simulink model "Temp_derating"  (R2021b)
settings: Solver=VariableStepAuto  StartTime=0.0  StopTime=600  RelTol=1e-3
undefined symbols (not defined in the file): sigbuilder_block
settings Model: Creator=mohamednasser  LastModifiedBy=mohamednasser

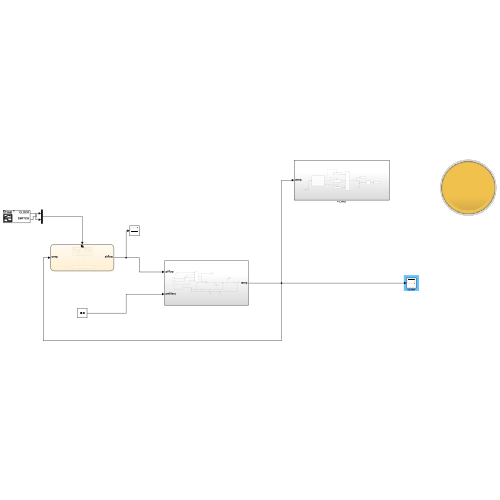
[thumbnail: Simulink's stored preview of the top-level diagram]
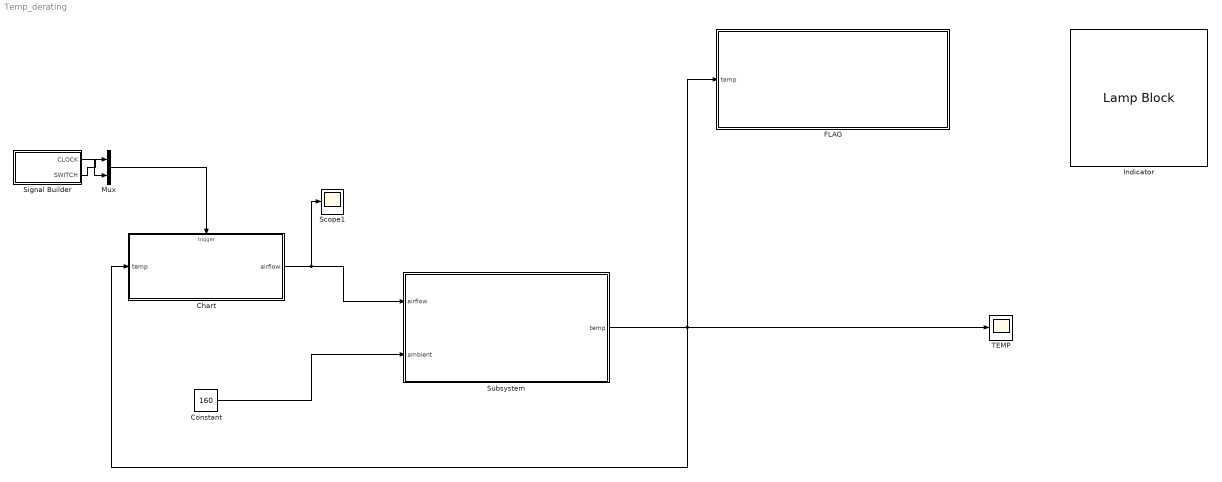
== system Temp_derating ==
  Chart : Stateflow chart  TreatAsAtomicUnit=on
  Constant : Constant  Value=160
  FLAG : Subsystem
  Indicator : LampBlock  LabelPosition=Hide
  Mux : Mux  Inputs=2
  Scope1 : Scope
  Signal Builder : Subsystem  Tag=STV Subsys  LoadFcn=sigbuilder_block('load');  StartFcn=sigbuilder_block('start');  StopFcn=sigbuilder_block('stop');  ClipboardFcn=sigbuilder_block('clipboard');  mask(Sigbuilder block){tuvar=[0:10]}
      mask help: Simulink:masks:SigbuilderBlock_MD
      mask init:
      | if ~strcmp(get_param(bdroot(gcbh),'SimulationStatus'),'stopped') tuvar = sigbuilder_block('maskInit'); end
      settings: CopyFcn=sigbuilder_block('copy');  DeleteFcn=sigbuilder_block('delete');  ModelCloseFcn=sigbuilder_block('modelClose');  PreSaveFcn=sigbuilder_block('preSave');  PauseFcn=sigbuilder_block('pause');  ContinueFcn=sigbuilder_block('continue');  NameChangeFcn=sigbuilder_block('namechange');  OpenFcn=sigbuilder_block('open',[377 114 550 400 ]);  CloseFcn=sigbuilder_block('close');
      mask Display: plot(0, 0, 100, 100,[2, 2, 32, 32, 2], [68, 8, 8, 68, 68],[32, 2], [38, 38], [32, 19, 2],[53, 60, 44], [32, 17, 17, 2],[16, 16, 31, 31]);txt = getActiveGroup(gcbh);text(2, 100, txt,'verticalAlignment', 'top');
  Subsystem : Subsystem
  TEMP : Scope
  wires:
  Subsystem/1(temp) -> TEMP/1, FLAG/1(temp), Chart/1(temp)
  Constant/1 -> Subsystem/2(ambient)
  Chart/1(airflow) -> Scope1/1, Subsystem/1(airflow)
  Mux/1 -> Chart/Trigger
  Signal Builder/1(CLOCK) -> Mux/2
  Signal Builder/2(SWITCH) -> Mux/1

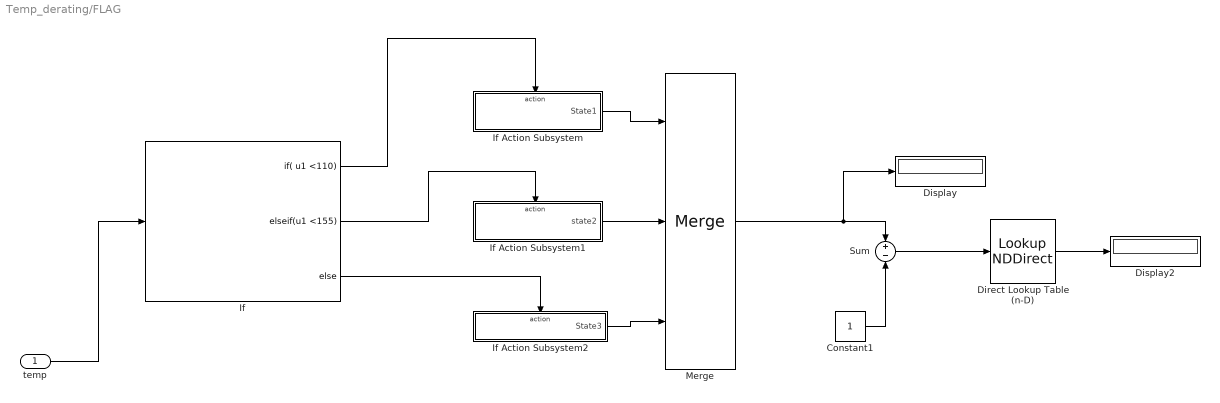
== system Temp_derating/FLAG ==
  temp : Inport
  Constant1 : Constant
  Direct Lookup Table (n-D) : LookupNDDirect  NumberOfTableDimensions=1  Table=[1 2 3]
  Display : Display
  Display2 : Display
  If : If  IfExpression=u1 <110  ElseIfExpressions=u1 <155
  If Action Subsystem : Subsystem  TreatAsAtomicUnit=on
  If Action Subsystem1 : Subsystem  TreatAsAtomicUnit=on
  If Action Subsystem2 : Subsystem  TreatAsAtomicUnit=on
  Merge : Merge  Inputs=3
  Sum : Sum  Inputs=+-
  wires:
  If/2 -> If Action Subsystem1/Action
  If/1 -> If Action Subsystem/Action
  Constant1/1 -> Sum/2
  Merge/1 -> Display/1, Sum/1
  If/3 -> If Action Subsystem2/Action
  If Action Subsystem1/1(state2) -> Merge/2
  Sum/1 -> Direct Lookup Table (n-D)/1
  If Action Subsystem/1(State1) -> Merge/1
  temp/1 -> If/1
  If Action Subsystem2/1(State3) -> Merge/3
  Direct Lookup Table (n-D)/1 -> Display2/1

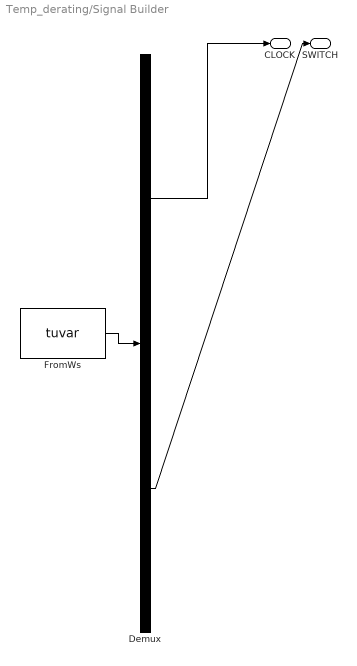
== system Temp_derating/Signal Builder ==
  Demux : Demux  Tag=STV Demux  Outputs=2
      settings: DisplayOption=none
  FromWs : FromWorkspace  Tag=STV FromWs  VariableName=tuvar
      SigBuilderData=|
      | common.afterFinalStr = 'Extrapolate'
      | common.sampleTime = 0
      | dataSet.timeRange = [0 600]
      | dataSet.name = 'Group 1'
      | sbobj.Groups.Name = 'Group 1'
      | sbobj.Groups.Signals(1).Name = 'CLOCK'
      | sbobj.Groups.Signals(1).XData = [0 0.5 0.5 1 1 1.5 1.5 2 2 2.5 2.5 3 ... (2400 elements, 1x2400)]
      | sbobj.Groups.Signals(1).YData = [2 2 0 0 2 2 0 0 2 2 0 0 ... (2400 elements, 1x2400)]
      | sbobj.Groups.Signals(2).Name = 'SWITCH'
      | sbobj.Groups.Signals(2).XData = [0 350 350 501 501 600]
      | sbobj.Groups.Signals(2).YData = [0 0 1 1 0 0]
      | sbobj.Groups.TimeRange = [0 600]
  CLOCK : Outport  Tag=STV Outport
  SWITCH : Outport  Tag=STV Outport  Port=2
  wires:
  FromWs/1 -> Demux/1
  Demux/1 -> CLOCK/1
  Demux/2 -> SWITCH/1

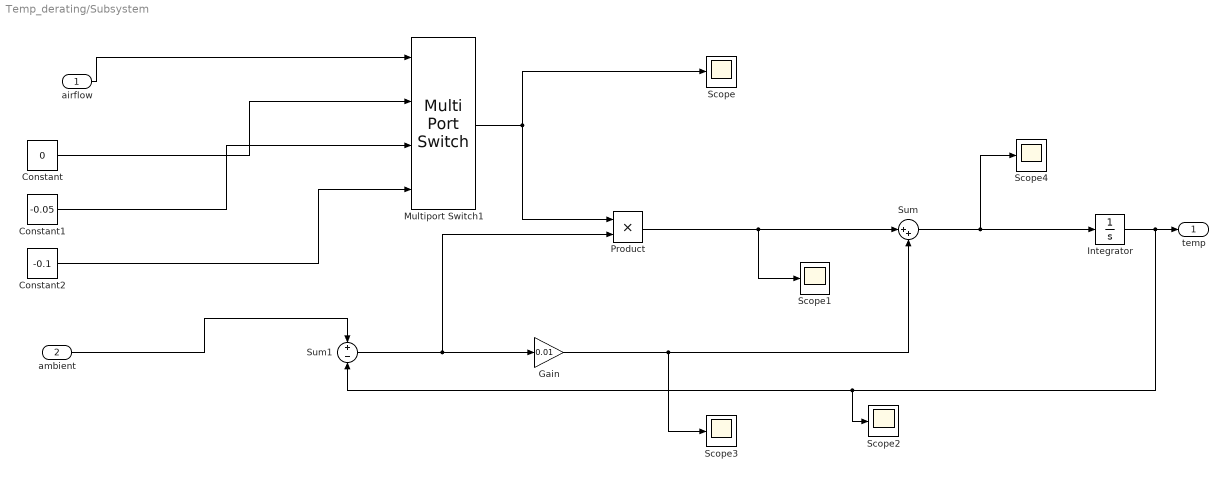
== system Temp_derating/Subsystem ==
  airflow : Inport
  ambient : Inport  Port=2
  Constant : Constant  Value=0
  Constant1 : Constant  Value=-0.05
  Constant2 : Constant  Value=-0.1
  Gain : Gain  Gain=0.01
  Integrator : Integrator  InitialCondition=70
  Multiport Switch1 : MultiPortSwitch  DataPortOrder=Zero-based contiguous  zeroidx=on
  Product : Product
  Scope{,1..4} (5 alike) : Scope
  Sum : Sum  Inputs=|++
  Sum1 : Sum  Inputs=+-
  temp : Outport
  wires:
  Constant/1 -> Multiport Switch1/2
  Constant2/1 -> Multiport Switch1/4
  airflow/1 -> Multiport Switch1/1
  Multiport Switch1/1 -> Product/1, Scope/1
  Constant1/1 -> Multiport Switch1/3
  ambient/1 -> Sum1/1
  Sum1/1 -> Product/2, Gain/1
  Sum/1 -> Scope4/1, Integrator/1
  Gain/1 -> Scope3/1, Sum/2
  Product/1 -> Scope1/1, Sum/1
  Integrator/1 -> Scope2/1, Sum1/2, temp/1

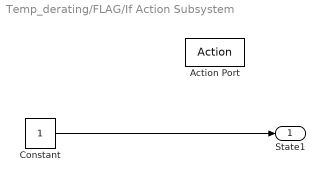
== system Temp_derating/FLAG/If Action Subsystem ==
  Action Port : ActionPort  ActionPortLabel=if( u1 <110)
  Constant : Constant
  State1 : Outport
  wires:
  Constant/1 -> State1/1

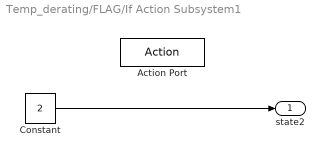
== system Temp_derating/FLAG/If Action Subsystem1 ==
  Action Port : ActionPort  ActionPortLabel=elseif(u1 <155)
  Constant : Constant  Value=2
  state2 : Outport
  wires:
  Constant/1 -> state2/1

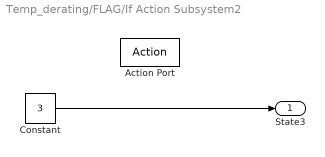
== system Temp_derating/FLAG/If Action Subsystem2 ==
  Action Port : ActionPort  ActionPortLabel=else
  Constant : Constant  Value=3
  State3 : Outport
  wires:
  Constant/1 -> State3/1

== stateflow chart Temp_derating/Chart ==
  settings: executeAtInitialization=1
  state Power_ON
    state Fan_1 [parallel]
      settings: executionOrder=1
      state On
      state Off
      (default) -> Power_ON.Fan_1.Off
      Power_ON.Fan_1.On -> Power_ON.Fan_1.Off : [temp < 120]
      Power_ON.Fan_1.Off -> Power_ON.Fan_1.On : [temp >= 120]
    state Fan_2 [parallel]
      settings: executionOrder=2
      state On
      state Off
      (default) -> Power_ON.Fan_2.Off
      Power_ON.Fan_2.On -> Power_ON.Fan_2.Off : [temp < 150]
      Power_ON.Fan_2.Off -> Power_ON.Fan_2.On : [temp>= 150]
    state Speed_Value [parallel]
      during: airflow = in(Fan_1.On) + in(Fan_2.On);
      settings: executionOrder=3
  state Power_OFF
    entry: airflow = 0;
  Power_OFF -> Power_ON : SWITCH
  Power_ON -> Power_OFF : SWITCH
  (default) -> Power_OFF
  data: temp input; airflow output uint8 [0..2]
  events: SWITCH input EITHER_EDGE_EVENT; CLOCK input EITHER_EDGE_EVENT
